simulink model "Appl_PaMemory_CtrlModel"  (R2018b)
settings: configuration reference "CodeConfig_10_ms" (kept outside this file)
undefined symbols (not defined in the file): CAL_PaMem_100MS, CAL_PaMem_90MS, D_ToleranceDistance, FALSE, TRUE
libraries: DareLib x89, simulink x1
(part 1 of 3)
settings Model: Creator=Administrator  LastModifiedBy=Administrator
settings ConfigSetRef: SourceLocation=Base Workspace

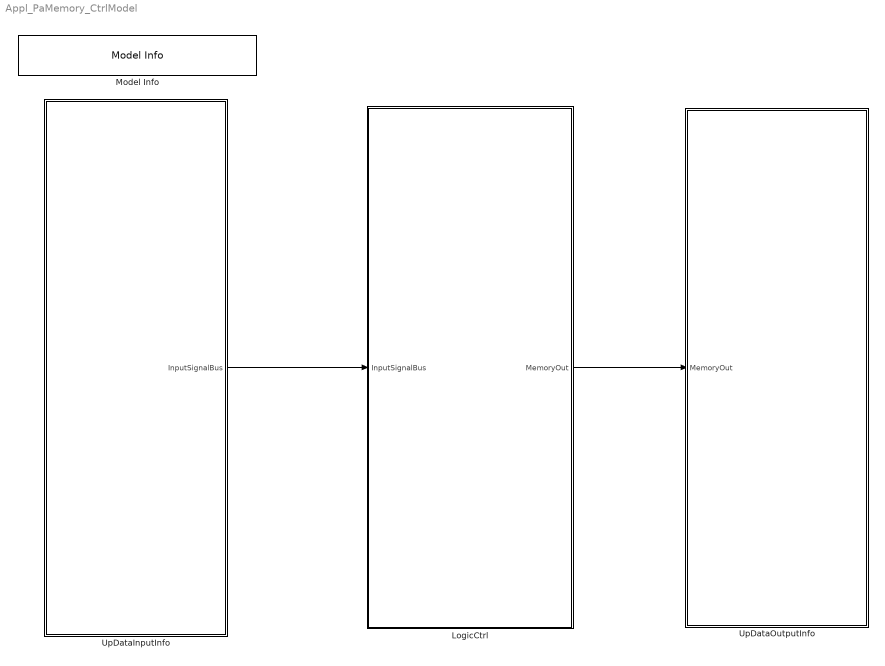
== system Appl_PaMemory_CtrlModel ==
  LogicCtrl : Subsystem  Priority=2  TreatAsAtomicUnit=on
      settings: RTWSystemCode=Nonreusable function  RTWFcnNameOpts=Use subsystem name
  Model Info : simulink/Model-Wide Utilities/Model Info  Frame=on  DisplayStringWithTags=Version：%<ModelVersion>  HorizontalTextAlignment=Center  LeftAlignmentValue=0.5
  UpDataInputInfo : Subsystem  Priority=1  TreatAsAtomicUnit=on
      settings: RTWSystemCode=Nonreusable function  RTWFcnNameOpts=Use subsystem name
  UpDataOutputInfo : Subsystem  Priority=3  TreatAsAtomicUnit=on
      settings: RTWSystemCode=Nonreusable function  RTWFcnNameOpts=Use subsystem name
  wires:
  LogicCtrl/1(MemoryOut) -> UpDataOutputInfo/1(MemoryOut)
  UpDataInputInfo/1(InputSignalBus) -> LogicCtrl/1(InputSignalBus)

== system Appl_PaMemory_CtrlModel/LogicCtrl ==
  InputSignalBus : Inport
  Bus Selector : BusSelector  OutputSignals=SeatMemBtn,CallMem,MemorySetPrecondition,MemoryRemindPrecondition,Rte_SignalBus.PaMem_HeightHallPosi,Rte_SignalBus.PaMem_LengthHallPosi,Rte_SignalBus.PaMem_BackHallPosi,Rte_SignalBus.PaMem_FrontHallPosi,Rte_SignalBus.PaMem_HeightAutoRunFlag,Rte_SignalBus.PaMem_LengthAutoRunFlag,Rte_SignalBus.PaMem_BackAutoRunFlag,Rte_SignalBus.PaMem_FrontAutoRunFlag,Rte_SignalBus.PaMem_AdjustEnable,Rte_SignalBus.PaMem_FRSeatPosMsg,Rte_SignalBus.PaMem_CurrentMoveType,Rte_SignalBus.PaMem_GetRecoverDefaultFlag,Rte_SignalBus.PaMem_HeightLockFault,Rte_SignalBus.PaMem_LengthLockFault,Rte_SignalBus.PaMem_BackLockFault,Rte_SignalBus.PaMem_FrontLockFault
  LocalAdjustCtrl : Subsystem  Description=加热逻辑处理
      settings: AttributesFormatString=%<Description>
  MainVent_OutputLvlSts : BusCreator  Inputs=13
  MemoryOut : Outport
  wires:
  InputSignalBus/1 -> Bus Selector/1  "InputSignalBus"
  MainVent_OutputLvlSts/1 -> MemoryOut/1  "MemoryOut"
  Bus Selector/1 -> LocalAdjustCtrl/1(SeatMemBtn)  "<SeatMemBtn>"
  Bus Selector/2 -> LocalAdjustCtrl/2(CallMem)  "<CallMem>"
  Bus Selector/3 -> LocalAdjustCtrl/3(MemorySetPrecondition)  "<MemorySetPrecondition>"
  Bus Selector/4 -> LocalAdjustCtrl/4(MemoryRemindPrecondition)  "<MemoryRemindPrecondition>"
  Bus Selector/5 -> LocalAdjustCtrl/5(PaMem_HeightHallPosi)  "<PaMem_HeightHallPosi>"
  Bus Selector/6 -> LocalAdjustCtrl/6(PaMem_LengthHallPosi)  "<PaMem_LengthHallPosi>"
  Bus Selector/7 -> LocalAdjustCtrl/7(PaMem_BackHallPosi)  "<PaMem_BackHallPosi>"
  Bus Selector/8 -> LocalAdjustCtrl/8(PaMem_FrontHallPosi)  "<PaMem_FrontHallPosi>"
  Bus Selector/9 -> LocalAdjustCtrl/9(PaMem_HeightAutoRunFlag)  "<PaMem_HeightAutoRunFlag>"
  Bus Selector/10 -> LocalAdjustCtrl/10(PaMem_LengthAutoRunFlag)  "<PaMem_LengthAutoRunFlag>"
  Bus Selector/11 -> LocalAdjustCtrl/11(PaMem_BackAutoRunFlag)  "<PaMem_BackAutoRunFlag>"
  Bus Selector/12 -> LocalAdjustCtrl/12(PaMem_FrontAutoRunFlag)  "<PaMem_FrontAutoRunFlag>"
  Bus Selector/13 -> LocalAdjustCtrl/13(PaMem_AdjustEnable)  "<PaMem_AdjustEnable>"
  Bus Selector/14 -> LocalAdjustCtrl/14(PaMem_FRSeatPosMsg)  "<PaMem_FRSeatPosMsg>"
  Bus Selector/15 -> LocalAdjustCtrl/15(PaMem_CurrentMoveType)  "<PaMem_CurrentMoveType>"
  Bus Selector/16 -> LocalAdjustCtrl/16(PaMem_GetRecoverDefaultFlag)  "<PaMem_GetRecoverDefaultFlag>"
  Bus Selector/17 -> LocalAdjustCtrl/17(PaMem_HeightLockFault)  "<PaMem_HeightLockFault>"
  Bus Selector/18 -> LocalAdjustCtrl/18(PaMem_LengthLockFault)  "<PaMem_LengthLockFault>"
  Bus Selector/19 -> LocalAdjustCtrl/19(PaMem_BackLockFault)  "<PaMem_BackLockFault>"
  Bus Selector/20 -> LocalAdjustCtrl/20(PaMem_FrontLockFault)  "<PaMem_FrontLockFault>"
  LocalAdjustCtrl/1(FRSeatMemSetSts) -> MainVent_OutputLvlSts/1
  LocalAdjustCtrl/2(MemSetStopReason) -> MainVent_OutputLvlSts/2
  LocalAdjustCtrl/3(FRSeatPosMsg) -> MainVent_OutputLvlSts/3
  LocalAdjustCtrl/4(SeatMemoryValidReq) -> MainVent_OutputLvlSts/4
  LocalAdjustCtrl/5(SeatHeightPosiReq) -> MainVent_OutputLvlSts/5
  LocalAdjustCtrl/6(SeatLengthPosiReq) -> MainVent_OutputLvlSts/6
  LocalAdjustCtrl/7(SeatBackPosiReq) -> MainVent_OutputLvlSts/7
  LocalAdjustCtrl/8(SeatFrontPosiReq) -> MainVent_OutputLvlSts/8
  LocalAdjustCtrl/9(MemCallStopReason) -> MainVent_OutputLvlSts/9
  LocalAdjustCtrl/10(SeatMem1StsFb) -> MainVent_OutputLvlSts/10
  LocalAdjustCtrl/11(SeatMem2StsFb) -> MainVent_OutputLvlSts/11
  LocalAdjustCtrl/12(SeatMem3StsFb) -> MainVent_OutputLvlSts/12
  LocalAdjustCtrl/13(PreMemRemindStop) -> MainVent_OutputLvlSts/13

== system Appl_PaMemory_CtrlModel/UpDataInputInfo ==
  InputSignalProcess : Subsystem  Description=数据处理
      settings: AttributesFormatString=%<Description>  RTWSystemCode=Nonreusable function  RTWFcnNameOpts=Use subsystem name
  RTE : Subsystem  Description=接口自动生成  TreatAsAtomicUnit=on
      settings: AttributesFormatString=%<Description>  RTWSystemCode=Nonreusable function  RTWFcnNameOpts=Use subsystem name
  InputSignalBus : Outport
  wires:
  RTE/1(RTE_Signal) -> InputSignalProcess/1(Rte_SignalBus)
  InputSignalProcess/1(InputSignalBus) -> InputSignalBus/1

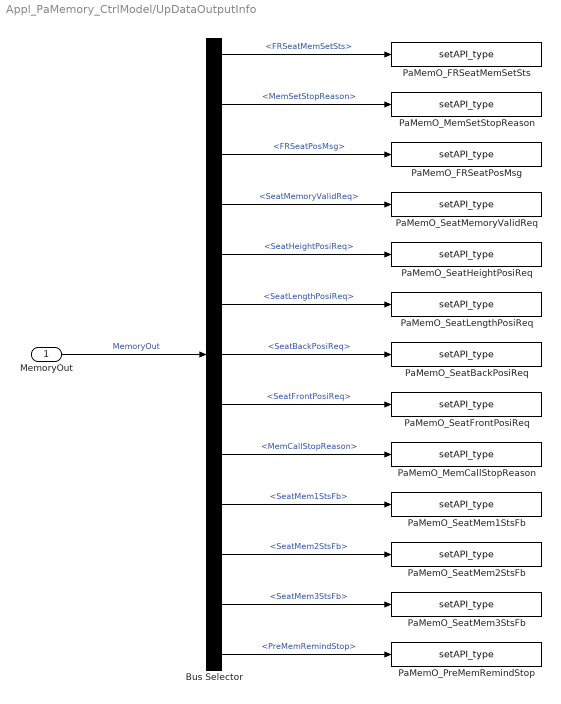
== system Appl_PaMemory_CtrlModel/UpDataOutputInfo ==
  MemoryOut : Inport
  Bus Selector : BusSelector  OutputSignals=FRSeatMemSetSts,MemSetStopReason,FRSeatPosMsg,SeatMemoryValidReq,SeatHeightPosiReq,SeatLengthPosiReq,SeatBackPosiReq,SeatFrontPosiReq,MemCallStopReason,SeatMem1StsFb,SeatMem2StsFb,SeatMem3StsFb,PreMemRemindStop
  PaMemO_FRSeatMemSetSts : DareLib/Dare/setAPI_type  g_funcname=CanTx_0x3B2_DSM_FRSeatMemStsAndMsg  g_param=""  g_type=uint8  g_enum=enMemSetFb  g_size=-1
      settings: AttributesFormatString=%<g_funcname>  SourceProductName=Dare Library
  PaMemO_FRSeatPosMsg : DareLib/Dare/setAPI_type  g_funcname=CanTx_0x3B2_DSM_FRSeatPosMsg  g_param=""  g_type=uint8  g_size=-1
      settings: AttributesFormatString=%<g_funcname>  SourceProductName=Dare Library
  PaMemO_MemCallStopReason : DareLib/Dare/setAPI_type  g_funcname=Rte_SetVfb_PaMemCallStopReason  g_param=""  g_type=uint8  g_enum=enMemStopCause  g_size=-1
      settings: AttributesFormatString=%<g_funcname>  SourceProductName=Dare Library
  PaMemO_MemSetStopReason : DareLib/Dare/setAPI_type  g_funcname=Rte_SetVfb_PaMemSetStopReason  g_param=""  g_type=uint8  g_enum=enMemStopCause  g_size=-1
      settings: AttributesFormatString=%<g_funcname>  SourceProductName=Dare Library
  PaMemO_PreMemRemindStop : DareLib/Dare/setAPI_type  g_funcname=Rte_SetVfb_PaPreMemRemindStop  g_param=""  g_type=uint8  g_enum=enMemStopCause  g_size=-1
      settings: AttributesFormatString=%<g_funcname>  SourceProductName=Dare Library
  PaMemO_SeatBackPosiReq : DareLib/Dare/setAPI_type  g_funcname=Rte_SetVfb_PaMemBackReqPosi  g_param=""  g_type=uint16  g_size=-1
      settings: AttributesFormatString=%<g_funcname>  SourceProductName=Dare Library
  PaMemO_SeatFrontPosiReq : DareLib/Dare/setAPI_type  g_funcname=Rte_SetVfb_PaMemFrontReqPosi  g_param=""  g_type=uint16  g_size=-1
      settings: AttributesFormatString=%<g_funcname>  SourceProductName=Dare Library
  PaMemO_SeatHeightPosiReq : DareLib/Dare/setAPI_type  g_funcname=Rte_SetVfb_PaMemHeightReqPosi  g_param=""  g_type=uint16  g_size=-1
      settings: AttributesFormatString=%<g_funcname>  SourceProductName=Dare Library
  PaMemO_SeatLengthPosiReq : DareLib/Dare/setAPI_type  g_funcname=Rte_SetVfb_PaMemLengthReqPosi  g_param=""  g_type=uint16  g_size=-1
      settings: AttributesFormatString=%<g_funcname>  SourceProductName=Dare Library
  PaMemO_SeatMem1StsFb : DareLib/Dare/setAPI_type  g_funcname=CanTx_0x3B2_DSM1_FRSeatMem1Sts  g_param=""  g_type=uint8  g_enum=enMemCallFb  g_size=-1
      settings: AttributesFormatString=%<g_funcname>  SourceProductName=Dare Library
  PaMemO_SeatMem2StsFb : DareLib/Dare/setAPI_type  g_funcname=CanTx_0x3B2_DSM2_FRSeatMem2Sts  g_param=""  g_type=uint8  g_enum=enMemCallFb  g_size=-1
      settings: AttributesFormatString=%<g_funcname>  SourceProductName=Dare Library
  PaMemO_SeatMem3StsFb : DareLib/Dare/setAPI_type  g_funcname=CanTx_0x3B2_DSM2_FRSeatMem3Sts  g_param=""  g_type=uint8  g_enum=enMemCallFb  g_size=-1
      settings: AttributesFormatString=%<g_funcname>  SourceProductName=Dare Library
  PaMemO_SeatMemoryValidReq : DareLib/Dare/setAPI_type  g_funcname=Rte_SetVfb_PaSeatMemoryValidReq  g_param=""  g_type=uint8  g_size=-1
      settings: AttributesFormatString=%<g_funcname>  SourceProductName=Dare Library
  wires:
  MemoryOut/1 -> Bus Selector/1  "MemoryOut"
  Bus Selector/2 -> PaMemO_MemSetStopReason/1  "<MemSetStopReason>"
  Bus Selector/1 -> PaMemO_FRSeatMemSetSts/1  "<FRSeatMemSetSts>"
  Bus Selector/3 -> PaMemO_FRSeatPosMsg/1  "<FRSeatPosMsg>"
  Bus Selector/4 -> PaMemO_SeatMemoryValidReq/1  "<SeatMemoryValidReq>"
  Bus Selector/5 -> PaMemO_SeatHeightPosiReq/1  "<SeatHeightPosiReq>"
  Bus Selector/6 -> PaMemO_SeatLengthPosiReq/1  "<SeatLengthPosiReq>"
  Bus Selector/7 -> PaMemO_SeatBackPosiReq/1  "<SeatBackPosiReq>"
  Bus Selector/8 -> PaMemO_SeatFrontPosiReq/1  "<SeatFrontPosiReq>"
  Bus Selector/9 -> PaMemO_MemCallStopReason/1  "<MemCallStopReason>"
  Bus Selector/10 -> PaMemO_SeatMem1StsFb/1  "<SeatMem1StsFb>"
  Bus Selector/11 -> PaMemO_SeatMem2StsFb/1  "<SeatMem2StsFb>"
  Bus Selector/12 -> PaMemO_SeatMem3StsFb/1  "<SeatMem3StsFb>"
  Bus Selector/13 -> PaMemO_PreMemRemindStop/1  "<PreMemRemindStop>"

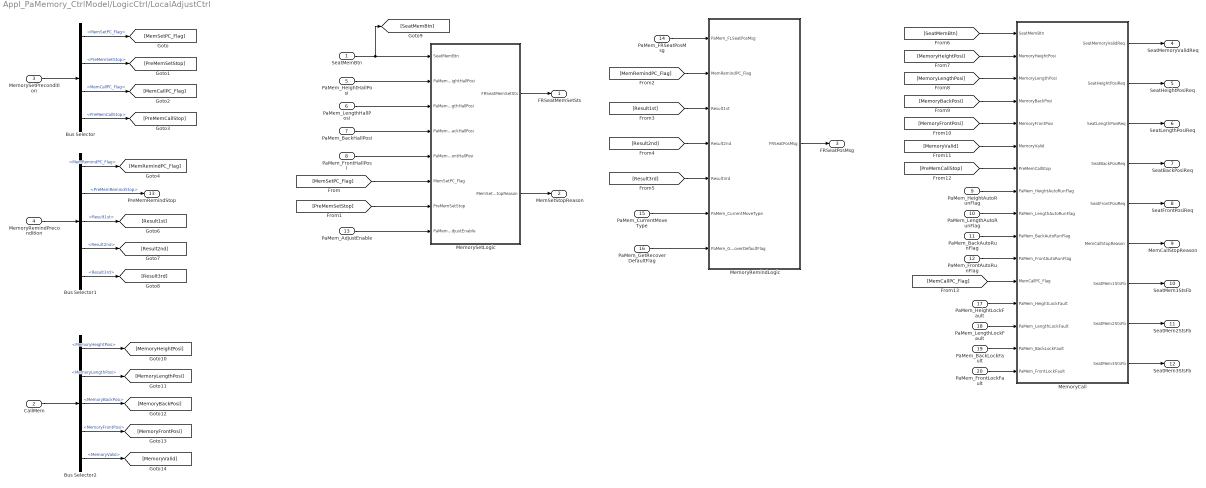
== system Appl_PaMemory_CtrlModel/LogicCtrl/LocalAdjustCtrl ==
  SeatMemBtn : Inport
  CallMem : Inport  Port=2
  MemorySetPrecondition : Inport  Port=3
  MemoryRemindPrecondition : Inport  Port=4
  PaMem_HeightHallPosi : Inport  Port=5
  PaMem_LengthHallPosi : Inport  Port=6
  PaMem_BackHallPosi : Inport  Port=7
  PaMem_FrontHallPosi : Inport  Port=8
  PaMem_HeightAutoRunFlag : Inport  Port=9
  PaMem_LengthAutoRunFlag : Inport  Port=10
  PaMem_BackAutoRunFlag : Inport  Port=11
  PaMem_FrontAutoRunFlag : Inport  Port=12
  PaMem_AdjustEnable : Inport  Port=13
  PaMem_FRSeatPosMsg : Inport  Port=14
  PaMem_CurrentMoveType : Inport  Port=15
  PaMem_GetRecoverDefaultFlag : Inport  Port=16
  PaMem_HeightLockFault : Inport  Port=17
  PaMem_LengthLockFault : Inport  Port=18
  PaMem_BackLockFault : Inport  Port=19
  PaMem_FrontLockFault : Inport  Port=20
  Bus Selector : BusSelector  OutputSignals=MemSetPC_Flag,PreMemSetStop,MemCallPC_Flag,PreMemCallStop
  Bus Selector1 : BusSelector  OutputSignals=MemRemindPC_Flag,PreMemRemindStop,Result1st,Result2nd,Result3rd
  Bus Selector2 : BusSelector  OutputSignals=MemoryHeightPosi,MemoryLengthPosi,MemoryBackPosi,MemoryFrontPosi,MemoryValid
  MemoryCall : Stateflow chart  TreatAsAtomicUnit=on
  MemoryRemindLogic : Stateflow chart  TreatAsAtomicUnit=on
  MemorySetLogic : Stateflow chart  TreatAsAtomicUnit=on
  FRSeatMemSetSts : Outport
  MemSetStopReason : Outport  Port=2
  FRSeatPosMsg : Outport  Port=3
  SeatMemoryValidReq : Outport  Port=4
  SeatHeightPosiReq : Outport  Port=5
  SeatLengthPosiReq : Outport  Port=6
  SeatBackPosiReq : Outport  Port=7
  SeatFrontPosiReq : Outport  Port=8
  MemCallStopReason : Outport  Port=9
  SeatMem1StsFb : Outport  Port=10
  SeatMem2StsFb : Outport  Port=11
  SeatMem3StsFb : Outport  Port=12
  PreMemRemindStop : Outport  Port=13
  wires:
  SeatMemBtn/1 -> [SeatMemBtn], MemorySetLogic/1(SeatMemBtn)
  PaMem_HeightHallPosi/1 -> MemorySetLogic/2(PaMem_HeightHallPosi)
  PaMem_LengthHallPosi/1 -> MemorySetLogic/3(PaMem_LengthHallPosi)
  PaMem_BackHallPosi/1 -> MemorySetLogic/4(PaMem_BackHallPosi)
  PaMem_FrontHallPosi/1 -> MemorySetLogic/5(PaMem_FrontHallPosi)
  MemorySetPrecondition/1 -> Bus Selector/1
  Bus Selector/1 -> [MemSetPC_Flag]  "<MemSetPC_Flag>"
  Bus Selector/2 -> [PreMemSetStop]  "<PreMemSetStop>"
  Bus Selector/3 -> [MemCallPC_Flag]  "<MemCallPC_Flag>"
  Bus Selector/4 -> [PreMemCallStop]  "<PreMemCallStop>"
  [MemSetPC_Flag] -> MemorySetLogic/6(MemSetPC_Flag)
  [PreMemSetStop] -> MemorySetLogic/7(PreMemSetStop)
  PaMem_AdjustEnable/1 -> MemorySetLogic/8(PaMem_AdjustEnable)
  MemoryRemindPrecondition/1 -> Bus Selector1/1
  Bus Selector1/4 -> [Result2nd]  "<Result2nd>"
  Bus Selector1/3 -> [Result1st]  "<Result1st>"
  Bus Selector1/5 -> [Result3rd]  "<Result3rd>"
  Bus Selector1/1 -> [MemRemindPC_Flag]  "<MemRemindPC_Flag>"
  PaMem_FRSeatPosMsg/1 -> MemoryRemindLogic/1(PaMem_FLSeatPosMsg)
  [MemRemindPC_Flag] -> MemoryRemindLogic/2(MemRemindPC_Flag)
  [Result1st] -> MemoryRemindLogic/3(Result1st)
  [Result2nd] -> MemoryRemindLogic/4(Result2nd)
  [Result3rd] -> MemoryRemindLogic/5(Result3rd)
  PaMem_CurrentMoveType/1 -> MemoryRemindLogic/6(PaMem_CurrentMoveType)
  PaMem_GetRecoverDefaultFlag/1 -> MemoryRemindLogic/7(PaMem_GetRecoverDefaultFlag)
  CallMem/1 -> Bus Selector2/1
  Bus Selector2/1 -> [MemoryHeightPosi]  "<MemoryHeightPosi>"
  Bus Selector2/2 -> [MemoryLengthPosi]  "<MemoryLengthPosi>"
  Bus Selector2/3 -> [MemoryBackPosi]  "<MemoryBackPosi>"
  Bus Selector2/4 -> [MemoryFrontPosi]  "<MemoryFrontPosi>"
  Bus Selector2/5 -> [MemoryValid]  "<MemoryValid>"
  [SeatMemBtn] -> MemoryCall/1(SeatMemBtn)
  [MemoryHeightPosi] -> MemoryCall/2(MemoryHeightPosi)
  [MemoryLengthPosi] -> MemoryCall/3(MemoryLengthPosi)
  [MemoryBackPosi] -> MemoryCall/4(MemoryBackPosi)
  [MemoryFrontPosi] -> MemoryCall/5(MemoryFrontPosi)
  [MemoryValid] -> MemoryCall/6(MemoryValid)
  [PreMemCallStop] -> MemoryCall/7(PreMemCallStop)
  PaMem_HeightAutoRunFlag/1 -> MemoryCall/8(PaMem_HeightAutoRunFlag)
  PaMem_LengthAutoRunFlag/1 -> MemoryCall/9(PaMem_LengthAutoRunFlag)
  PaMem_BackAutoRunFlag/1 -> MemoryCall/10(PaMem_BackAutoRunFlag)
  PaMem_FrontAutoRunFlag/1 -> MemoryCall/11(PaMem_FrontAutoRunFlag)
  [MemCallPC_Flag] -> MemoryCall/12(MemCallPC_Flag)
  PaMem_FrontLockFault/1 -> MemoryCall/16(PaMem_FrontLockFault)
  PaMem_BackLockFault/1 -> MemoryCall/15(PaMem_BackLockFault)
  PaMem_LengthLockFault/1 -> MemoryCall/14(PaMem_LengthLockFault)
  PaMem_HeightLockFault/1 -> MemoryCall/13(PaMem_HeightLockFault)
  MemorySetLogic/1(FRSeatMemSetSts) -> FRSeatMemSetSts/1
  MemorySetLogic/2(MemSetStopReason) -> MemSetStopReason/1
  MemoryRemindLogic/1(FRSeatPosMsg) -> FRSeatPosMsg/1
  MemoryCall/1(SeatMemoryValidReq) -> SeatMemoryValidReq/1
  MemoryCall/2(SeatHeightPosiReq) -> SeatHeightPosiReq/1
  MemoryCall/3(SeatLengthPosiReq) -> SeatLengthPosiReq/1
  MemoryCall/4(SeatBackPosiReq) -> SeatBackPosiReq/1
  MemoryCall/5(SeatFrontPosiReq) -> SeatFrontPosiReq/1
  MemoryCall/6(MemCallStopReason) -> MemCallStopReason/1
  MemoryCall/7(SeatMem1StsFb) -> SeatMem1StsFb/1
  MemoryCall/8(SeatMem2StsFb) -> SeatMem2StsFb/1
  MemoryCall/9(SeatMem3StsFb) -> SeatMem3StsFb/1
  Bus Selector1/2 -> PreMemRemindStop/1  "<PreMemRemindStop>"

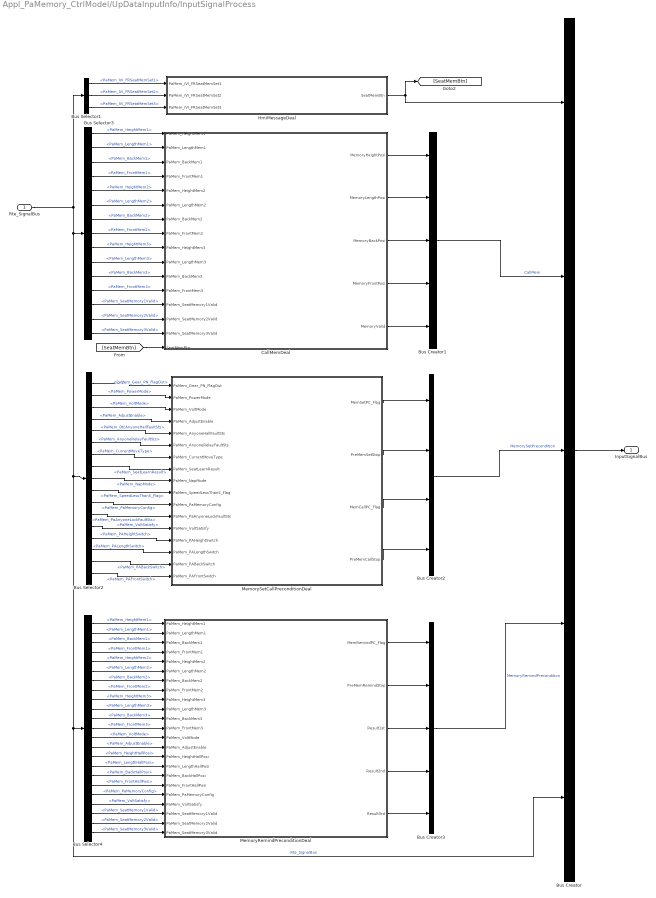
== system Appl_PaMemory_CtrlModel/UpDataInputInfo/InputSignalProcess ==
  Rte_SignalBus : Inport
  Bus Creator : BusCreator  Inputs=5
  Bus Creator1 : BusCreator  Inputs=5
  Bus Creator2 : BusCreator  Inputs=4
  Bus Creator3 : BusCreator  Inputs=5
  Bus Selector1 : BusSelector  OutputSignals=PaMem_IVI_FRSeatMemSet1,PaMem_IVI_FRSeatMemSet2,PaMem_IVI_FRSeatMemSet3
  Bus Selector2 : BusSelector  OutputSignals=PaMem_Gear_PN_FlagOut,PaMem_PowerMode,PaMem_VoltMode,PaMem_AdjustEnable,PaMem_DtcAnyoneHallFaultSts,PaMem_AnyoneRelayFaultSts,PaMem_CurrentMoveType,PaMem_SeatLearnResult,PaMem_NapMode,PaMem_SpeedLessThan5_Flag,PaMem_PaMemoryConfig,PaMem_PaAnyoneLockFaultSts,PaMem_VoltSatisfy,PaMem_PAHeightSwitch,PaMem_PALengthSwitch,PaMem_PABackSwitch,PaMem_PAFrontSwitch
  Bus Selector3 : BusSelector  OutputSignals=PaMem_HeightMem1,PaMem_LengthMem1,PaMem_BackMem1,PaMem_FrontMem1,PaMem_HeightMem2,PaMem_LengthMem2,PaMem_BackMem2,PaMem_FrontMem2,PaMem_HeightMem3,PaMem_LengthMem3,PaMem_BackMem3,PaMem_FrontMem3,PaMem_SeatMemory1Valid,PaMem_SeatMemory2Valid,PaMem_SeatMemory3Valid
  Bus Selector4 : BusSelector  OutputSignals=PaMem_HeightMem1,PaMem_LengthMem1,PaMem_BackMem1,PaMem_FrontMem1,PaMem_HeightMem2,PaMem_LengthMem2,PaMem_BackMem2,PaMem_FrontMem2,PaMem_HeightMem3,PaMem_LengthMem3,PaMem_BackMem3,PaMem_FrontMem3,PaMem_VoltMode,PaMem_AdjustEnable,PaMem_HeightHallPosi,PaMem_LengthHallPosi,PaMem_BackHallPosi,PaMem_FrontHallPosi,PaMem_PaMemoryConfig,PaMem_VoltSatisfy,PaMem_SeatMemory1Valid,PaMem_SeatMemory2Valid,PaMem_SeatMemory3Valid
  CallMemDeal : Subsystem  Description=记忆调用位置处理
      settings: AttributesFormatString=%<Description>
  HmiMessageDeal : Subsystem  Description=记忆报文处理
      settings: AttributesFormatString=%<Description>
  MemoryRemindPreconditionDeal : Subsystem  Description=记忆提示前置条件处理
      settings: AttributesFormatString=%<Description>
  MemorySetCallPreconditionDeal : Subsystem  Description=记忆设置与调用前置条件处理
      settings: AttributesFormatString=%<Description>
  InputSignalBus : Outport
  wires:
  Bus Creator/1 -> InputSignalBus/1
  Rte_SignalBus/1 -> Bus Selector4/1, Bus Creator/5, Bus Selector2/1, Bus Selector3/1, Bus Selector1/1  "Rte_SignalBus"
  HmiMessageDeal/1(SeatMemBtn) -> [SeatMemBtn], Bus Creator/1
  Bus Selector1/1 -> HmiMessageDeal/1(PaMem_IVI_FRSeatMemSet1)  "<PaMem_IVI_FRSeatMemSet1>"
  Bus Selector1/2 -> HmiMessageDeal/2(PaMem_IVI_FRSeatMemSet2)  "<PaMem_IVI_FRSeatMemSet2>"
  Bus Selector1/3 -> HmiMessageDeal/3(PaMem_IVI_FRSeatMemSet3)  "<PaMem_IVI_FRSeatMemSet3>"
  Bus Selector3/1 -> CallMemDeal/1(PaMem_HeightMem1)  "<PaMem_HeightMem1>"
  Bus Selector3/2 -> CallMemDeal/2(PaMem_LengthMem1)  "<PaMem_LengthMem1>"
  Bus Selector3/3 -> CallMemDeal/3(PaMem_BackMem1)  "<PaMem_BackMem1>"
  Bus Selector3/4 -> CallMemDeal/4(PaMem_FrontMem1)  "<PaMem_FrontMem1>"
  Bus Selector3/5 -> CallMemDeal/5(PaMem_HeightMem2)  "<PaMem_HeightMem2>"
  Bus Selector3/6 -> CallMemDeal/6(PaMem_LengthMem2)  "<PaMem_LengthMem2>"
  Bus Selector3/7 -> CallMemDeal/7(PaMem_BackMem2)  "<PaMem_BackMem2>"
  Bus Selector3/8 -> CallMemDeal/8(PaMem_FrontMem2)  "<PaMem_FrontMem2>"
  Bus Selector3/9 -> CallMemDeal/9(PaMem_HeightMem3)  "<PaMem_HeightMem3>"
  Bus Selector3/10 -> CallMemDeal/10(PaMem_LengthMem3)  "<PaMem_LengthMem3>"
  Bus Selector3/11 -> CallMemDeal/11(PaMem_BackMem3)  "<PaMem_BackMem3>"
  Bus Selector3/12 -> CallMemDeal/12(PaMem_FrontMem3)  "<PaMem_FrontMem3>"
  [SeatMemBtn] -> CallMemDeal/16(SeatMemBtn)
  CallMemDeal/1(MemoryHeightPosi) -> Bus Creator1/1
  CallMemDeal/2(MemoryLengthPosi) -> Bus Creator1/2
  CallMemDeal/3(MemoryBackPosi) -> Bus Creator1/3
  CallMemDeal/4(MemoryFrontPosi) -> Bus Creator1/4
  CallMemDeal/5(MemoryValid) -> Bus Creator1/5
  Bus Selector2/2 -> MemorySetCallPreconditionDeal/2(PaMem_PowerMode)  "<PaMem_PowerMode>"
  Bus Selector2/1 -> MemorySetCallPreconditionDeal/1(PaMem_Gear_PN_FlagOut)  "<PaMem_Gear_PN_FlagOut>"
  Bus Selector2/3 -> MemorySetCallPreconditionDeal/3(PaMem_VoltMode)  "<PaMem_VoltMode>"
  Bus Selector2/4 -> MemorySetCallPreconditionDeal/4(PaMem_AdjustEnable)  "<PaMem_AdjustEnable>"
  Bus Selector2/5 -> MemorySetCallPreconditionDeal/5(PaMem_AnyoneHallFaultSts)  "<PaMem_DtcAnyoneHallFaultSts>"
  Bus Selector2/7 -> MemorySetCallPreconditionDeal/7(PaMem_CurrentMoveType)  "<PaMem_CurrentMoveType>"
  Bus Selector2/8 -> MemorySetCallPreconditionDeal/8(PaMem_SeatLearnResult)  "<PaMem_SeatLearnResult>"
  Bus Selector2/9 -> MemorySetCallPreconditionDeal/9(PaMem_NapMode)  "<PaMem_NapMode>"
  Bus Selector2/6 -> MemorySetCallPreconditionDeal/6(PaMem_AnyoneRelayFaultSts)  "<PaMem_AnyoneRelayFaultSts>"
  Bus Selector4/5 -> MemoryRemindPreconditionDeal/5(PaMem_HeightMem2)  "<PaMem_HeightMem2>"
  Bus Selector4/4 -> MemoryRemindPreconditionDeal/4(PaMem_FrontMem1)  "<PaMem_FrontMem1>"
  Bus Selector4/6 -> MemoryRemindPreconditionDeal/6(PaMem_LengthMem2)  "<PaMem_LengthMem2>"
  Bus Selector4/3 -> MemoryRemindPreconditionDeal/3(PaMem_BackMem1)  "<PaMem_BackMem1>"
  Bus Selector4/7 -> MemoryRemindPreconditionDeal/7(PaMem_BackMem2)  "<PaMem_BackMem2>"
  Bus Selector4/2 -> MemoryRemindPreconditionDeal/2(PaMem_LengthMem1)  "<PaMem_LengthMem1>"
  Bus Selector4/8 -> MemoryRemindPreconditionDeal/8(PaMem_FrontMem2)  "<PaMem_FrontMem2>"
  Bus Selector4/1 -> MemoryRemindPreconditionDeal/1(PaMem_HeightMem1)  "<PaMem_HeightMem1>"
  Bus Selector4/9 -> MemoryRemindPreconditionDeal/9(PaMem_HeightMem3)  "<PaMem_HeightMem3>"
  Bus Selector4/10 -> MemoryRemindPreconditionDeal/10(PaMem_LengthMem3)  "<PaMem_LengthMem3>"
  Bus Selector4/11 -> MemoryRemindPreconditionDeal/11(PaMem_BackMem3)  "<PaMem_BackMem3>"
  Bus Selector4/12 -> MemoryRemindPreconditionDeal/12(PaMem_FrontMem3)  "<PaMem_FrontMem3>"
  Bus Selector4/13 -> MemoryRemindPreconditionDeal/13(PaMem_VoltMode)  "<PaMem_VoltMode>"
  Bus Selector4/14 -> MemoryRemindPreconditionDeal/14(PaMem_AdjustEnable)  "<PaMem_AdjustEnable>"
  Bus Selector4/15 -> MemoryRemindPreconditionDeal/15(PaMem_HeightHallPosi)  "<PaMem_HeightHallPosi>"
  Bus Selector4/16 -> MemoryRemindPreconditionDeal/16(PaMem_LengthHallPosi)  "<PaMem_LengthHallPosi>"
  Bus Selector4/17 -> MemoryRemindPreconditionDeal/17(PaMem_BackHallPosi)  "<PaMem_BackHallPosi>"
  Bus Selector4/18 -> MemoryRemindPreconditionDeal/18(PaMem_FrontHallPosi)  "<PaMem_FrontHallPosi>"
  MemorySetCallPreconditionDeal/1(MemSetPC_Flag) -> Bus Creator2/1
  MemorySetCallPreconditionDeal/2(PreMemSetStop) -> Bus Creator2/2
  MemorySetCallPreconditionDeal/3(MemCallPC_Flag) -> Bus Creator2/3
  MemorySetCallPreconditionDeal/4(PreMemCallStop) -> Bus Creator2/4
  MemoryRemindPreconditionDeal/2(PreMemRemindStop) -> Bus Creator3/2
  MemoryRemindPreconditionDeal/1(MemRemindPC_Flag) -> Bus Creator3/1
  MemoryRemindPreconditionDeal/3(Result1st) -> Bus Creator3/3
  MemoryRemindPreconditionDeal/4(Result2nd) -> Bus Creator3/4
  MemoryRemindPreconditionDeal/5(Result3rd) -> Bus Creator3/5
  Bus Creator1/1 -> Bus Creator/2  "CallMem"
  Bus Creator2/1 -> Bus Creator/3  "MemorySetPrecondition"
  Bus Creator3/1 -> Bus Creator/4  "MemoryRemindPrecondition"
  Bus Selector3/13 -> CallMemDeal/13(PaMem_SeatMemory1Valid)  "<PaMem_SeatMemory1Valid>"
  Bus Selector3/14 -> CallMemDeal/14(PaMem_SeatMemory2Valid)  "<PaMem_SeatMemory2Valid>"
  Bus Selector3/15 -> CallMemDeal/15(PaMem_SeatMemory3Valid)  "<PaMem_SeatMemory3Valid>"
  Bus Selector2/10 -> MemorySetCallPreconditionDeal/10(PaMem_SpeedLessThan5_Flag)  "<PaMem_SpeedLessThan5_Flag>"
  Bus Selector2/11 -> MemorySetCallPreconditionDeal/11(PaMem_PaMemoryConfig)  "<PaMem_PaMemoryConfig>"
  Bus Selector4/19 -> MemoryRemindPreconditionDeal/19(PaMem_PaMemoryConfig)  "<PaMem_PaMemoryConfig>"
  Bus Selector2/12 -> MemorySetCallPreconditionDeal/12(PaMem_PaAnyoneLockFaultSts)  "<PaMem_PaAnyoneLockFaultSts>"
  Bus Selector2/13 -> MemorySetCallPreconditionDeal/13(PaMem_VoltSatisfy)  "<PaMem_VoltSatisfy>"
  Bus Selector4/20 -> MemoryRemindPreconditionDeal/20(PaMem_VoltSatisfy)  "<PaMem_VoltSatisfy>"
  Bus Selector4/21 -> MemoryRemindPreconditionDeal/21(PaMem_SeatMemory1Valid)  "<PaMem_SeatMemory1Valid>"
  Bus Selector4/22 -> MemoryRemindPreconditionDeal/22(PaMem_SeatMemory2Valid)  "<PaMem_SeatMemory2Valid>"
  Bus Selector4/23 -> MemoryRemindPreconditionDeal/23(PaMem_SeatMemory3Valid)  "<PaMem_SeatMemory3Valid>"
  Bus Selector2/14 -> MemorySetCallPreconditionDeal/14(PaMem_PAHeightSwitch)  "<PaMem_PAHeightSwitch>"
  Bus Selector2/15 -> MemorySetCallPreconditionDeal/15(PaMem_PALengthSwitch)  "<PaMem_PALengthSwitch>"
  Bus Selector2/16 -> MemorySetCallPreconditionDeal/16(PaMem_PABackSwitch)  "<PaMem_PABackSwitch>"
  Bus Selector2/17 -> MemorySetCallPreconditionDeal/17(PaMem_PAFrontSwitch)  "<PaMem_PAFrontSwitch>"

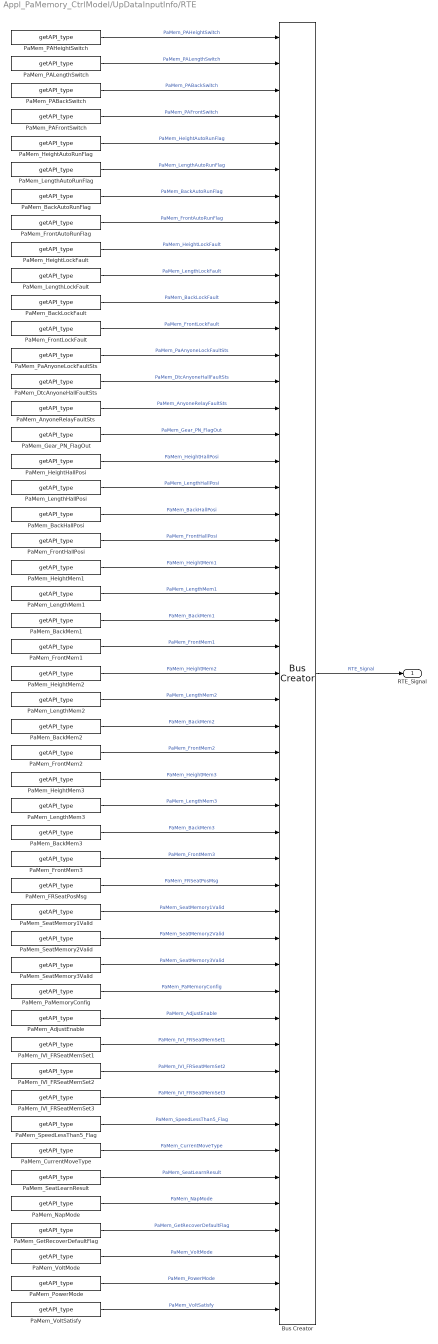
== system Appl_PaMemory_CtrlModel/UpDataInputInfo/RTE ==
  Bus Creator : BusCreator  Inputs=49
  PaMem_AdjustEnable : DareLib/Dare/getAPI_type  g_funcname=Srvl_GetMemIndexDataU8  g_param=EN_MemIndex_PaAdjustConfig  g_type=uint8  g_size=-1
      settings: AttributesFormatString=%<g_funcname>  SourceProductName=Dare Library
  PaMem_AnyoneRelayFaultSts : DareLib/Dare/getAPI_type  g_funcname=Rte_GetVfb_PaAnyoneRelayAdheErr  g_param=""  g_type=uint8  g_enum=enSeatMotorRunType  g_size=-1
      settings: AttributesFormatString=%<g_funcname>  SourceProductName=Dare Library
  PaMem_BackAutoRunFlag : DareLib/Dare/getAPI_type  g_funcname=Rte_GetVfb_PaBackAutoRunFlag  g_param=""  g_type=uint8  g_enum=enSeatAutoRunSts  g_size=-1
      settings: AttributesFormatString=%<g_funcname>  SourceProductName=Dare Library
  PaMem_BackHallPosi : DareLib/Dare/getAPI_type  g_funcname=Cdd_GetCurrentHallCnt  g_param=EN_PassengerBack  g_type=uint16  g_size=-1
      settings: AttributesFormatString=%<g_funcname>  SourceProductName=Dare Library
  PaMem_BackLockFault : DareLib/Dare/getAPI_type  g_funcname=Rte_GetVfb_PaBackStallErr  g_param=""  g_type=uint8  g_size=-1
      settings: AttributesFormatString=%<g_funcname>  SourceProductName=Dare Library
  PaMem_BackMem1 : DareLib/Dare/getAPI_type  g_funcname=Srvl_GetMemIndexDataU16  g_param=EN_MemIndex_PaMem1_Back  g_type=uint16  g_size=-1
      settings: AttributesFormatString=%<g_funcname>  SourceProductName=Dare Library
  PaMem_BackMem2 : DareLib/Dare/getAPI_type  g_funcname=Srvl_GetMemIndexDataU16  g_param=EN_MemIndex_PaMem2_Back  g_type=uint16  g_size=-1
      settings: AttributesFormatString=%<g_funcname>  SourceProductName=Dare Library
  PaMem_BackMem3 : DareLib/Dare/getAPI_type  g_funcname=Srvl_GetMemIndexDataU16  g_param=EN_MemIndex_PaMem3_Back  g_type=uint16  g_size=-1
      settings: AttributesFormatString=%<g_funcname>  SourceProductName=Dare Library
  PaMem_CurrentMoveType : DareLib/Dare/getAPI_type  g_funcname=Rte_GetVfb_PaMoveType  g_param=""  g_type=uint8  g_size=-1
      settings: AttributesFormatString=%<g_funcname>  SourceProductName=Dare Library
  PaMem_DtcAnyoneHallFaultSts : DareLib/Dare/getAPI_type  g_funcname=Rte_GetVfb_PaAnyoneDTCHallErr  g_param=""  g_type=uint8  g_size=-1
      settings: AttributesFormatString=%<g_funcname>  SourceProductName=Dare Library
  PaMem_FRSeatPosMsg : DareLib/Dare/getAPI_type  g_funcname=Srvl_GetMemIndexDataU8  g_param=EN_MemIndex_FRSeatPosMsg  g_type=uint8  g_size=-1
      settings: AttributesFormatString=%<g_funcname>  SourceProductName=Dare Library
  PaMem_FrontAutoRunFlag : DareLib/Dare/getAPI_type  g_funcname=Rte_GetVfb_PaFrontAutoRunFlag  g_param=""  g_type=uint8  g_enum=enSeatAutoRunSts  g_size=-1
      settings: AttributesFormatString=%<g_funcname>  SourceProductName=Dare Library
  PaMem_FrontHallPosi : DareLib/Dare/getAPI_type  g_funcname=Cdd_GetCurrentHallCnt  g_param=EN_PaResever_2  g_type=uint16  g_size=-1
      settings: AttributesFormatString=%<g_funcname>  SourceProductName=Dare Library
  PaMem_FrontLockFault : DareLib/Dare/getAPI_type  g_funcname=Rte_GetVfb_PaFrontStallErr  g_param=""  g_type=uint8  g_size=-1
      settings: AttributesFormatString=%<g_funcname>  SourceProductName=Dare Library
  PaMem_FrontMem1 : DareLib/Dare/getAPI_type  g_funcname=Srvl_GetMemIndexDataU16  g_param=EN_MemIndex_PaMem1_Front  g_type=uint16  g_size=-1
      settings: AttributesFormatString=%<g_funcname>  SourceProductName=Dare Library
  PaMem_FrontMem2 : DareLib/Dare/getAPI_type  g_funcname=Srvl_GetMemIndexDataU16  g_param=EN_MemIndex_PaMem2_Front  g_type=uint16  g_size=-1
      settings: AttributesFormatString=%<g_funcname>  SourceProductName=Dare Library
  PaMem_FrontMem3 : DareLib/Dare/getAPI_type  g_funcname=Srvl_GetMemIndexDataU16  g_param=EN_MemIndex_PaMem3_Front  g_type=uint16  g_size=-1
      settings: AttributesFormatString=%<g_funcname>  SourceProductName=Dare Library
  PaMem_Gear_PN_FlagOut : DareLib/Dare/getAPI_type  g_funcname=Rte_GetCAN_Gear_PN_Flag  g_param=""  g_type=uint8  g_size=-1
      settings: AttributesFormatString=%<g_funcname>  SourceProductName=Dare Library
  PaMem_GetRecoverDefaultFlag : DareLib/Dare/getAPI_type  g_funcname=GetRecoverDefaultFlag  g_param=""  g_type=uint16  g_size=-1
      settings: AttributesFormatString=%<g_funcname>  SourceProductName=Dare Library
  PaMem_HeightAutoRunFlag : DareLib/Dare/getAPI_type  g_funcname=Rte_GetVfb_PaHeightAutoRunFlag  g_param=""  g_type=uint8  g_enum=enSeatAutoRunSts  g_size=-1
      settings: AttributesFormatString=%<g_funcname>  SourceProductName=Dare Library
  PaMem_HeightHallPosi : DareLib/Dare/getAPI_type  g_funcname=Cdd_GetCurrentHallCnt  g_param=EN_PaResever_1  g_type=uint16  g_size=-1
      settings: AttributesFormatString=%<g_funcname>  SourceProductName=Dare Library
  PaMem_HeightLockFault : DareLib/Dare/getAPI_type  g_funcname=Rte_GetVfb_PaHeightStallErr  g_param=""  g_type=uint8  g_size=-1
      settings: AttributesFormatString=%<g_funcname>  SourceProductName=Dare Library
  PaMem_HeightMem1 : DareLib/Dare/getAPI_type  g_funcname=Srvl_GetMemIndexDataU16  g_param=EN_MemIndex_PaMem1_Height  g_type=uint16  g_size=-1
      settings: AttributesFormatString=%<g_funcname>  SourceProductName=Dare Library
  PaMem_HeightMem2 : DareLib/Dare/getAPI_type  g_funcname=Srvl_GetMemIndexDataU16  g_param=EN_MemIndex_PaMem2_Height  g_type=uint16  g_size=-1
      settings: AttributesFormatString=%<g_funcname>  SourceProductName=Dare Library
  PaMem_HeightMem3 : DareLib/Dare/getAPI_type  g_funcname=Srvl_GetMemIndexDataU16  g_param=EN_MemIndex_PaMem3_Height  g_type=uint16  g_size=-1
      settings: AttributesFormatString=%<g_funcname>  SourceProductName=Dare Library
  PaMem_IVI_FRSeatMemSet1 : DareLib/Dare/getAPI_type  g_funcname=CanRx_0x351_IVI_FRSeatMemSet1  g_param=""  g_type=uint8  g_enum=enMemSet  g_size=-1
      settings: AttributesFormatString=%<g_funcname>  SourceProductName=Dare Library
  PaMem_IVI_FRSeatMemSet2 : DareLib/Dare/getAPI_type  g_funcname=CanRx_0x351_IVI_FRSeatMemSet2  g_param=""  g_type=uint8  g_enum=enMemSet  g_size=-1
      settings: AttributesFormatString=%<g_funcname>  SourceProductName=Dare Library
  PaMem_IVI_FRSeatMemSet3 : DareLib/Dare/getAPI_type  g_funcname=CanRx_0x351_IVI_FRSeatMemSet3  g_param=""  g_type=uint8  g_enum=enMemSet  g_size=-1
      settings: AttributesFormatString=%<g_funcname>  SourceProductName=Dare Library
  PaMem_LengthAutoRunFlag : DareLib/Dare/getAPI_type  g_funcname=Rte_GetVfb_PaLengthAutoRunFlag  g_param=""  g_type=uint8  g_enum=enSeatAutoRunSts  g_size=-1
      settings: AttributesFormatString=%<g_funcname>  SourceProductName=Dare Library
  PaMem_LengthHallPosi : DareLib/Dare/getAPI_type  g_funcname=Cdd_GetCurrentHallCnt  g_param=EN_PassengerLength  g_type=uint16  g_size=-1
      settings: AttributesFormatString=%<g_funcname>  SourceProductName=Dare Library
  PaMem_LengthLockFault : DareLib/Dare/getAPI_type  g_funcname=Rte_GetVfb_PaLengthStallErr  g_param=""  g_type=uint8  g_size=-1
      settings: AttributesFormatString=%<g_funcname>  SourceProductName=Dare Library
  PaMem_LengthMem1 : DareLib/Dare/getAPI_type  g_funcname=Srvl_GetMemIndexDataU16  g_param=EN_MemIndex_PaMem1_Length  g_type=uint16  g_size=-1
      settings: AttributesFormatString=%<g_funcname>  SourceProductName=Dare Library
  PaMem_LengthMem2 : DareLib/Dare/getAPI_type  g_funcname=Srvl_GetMemIndexDataU16  g_param=EN_MemIndex_PaMem2_Length  g_type=uint16  g_size=-1
      settings: AttributesFormatString=%<g_funcname>  SourceProductName=Dare Library
  PaMem_LengthMem3 : DareLib/Dare/getAPI_type  g_funcname=Srvl_GetMemIndexDataU16  g_param=EN_MemIndex_PaMem3_Length  g_type=uint16  g_size=-1
      settings: AttributesFormatString=%<g_funcname>  SourceProductName=Dare Library
  PaMem_NapMode : DareLib/Dare/getAPI_type  g_funcname=Rte_GetVfb_NapMode  g_param=""  g_type=uint8  g_enum=enNapMode  g_size=-1
      settings: AttributesFormatString=%<g_funcname>  SourceProductName=Dare Library
  PaMem_PABackSwitch : DareLib/Dare/getAPI_type  g_funcname=Rte_GetVfb_PaBackSwitchCmd  g_param=""  g_type=uint8  g_size=-1
      settings: AttributesFormatString=%<g_funcname>  SourceProductName=Dare Library
  PaMem_PAFrontSwitch : DareLib/Dare/getAPI_type  g_funcname=Rte_GetVfb_PaFrontSwitchCmd  g_param=""  g_type=uint8  g_size=-1
      settings: AttributesFormatString=%<g_funcname>  SourceProductName=Dare Library
  PaMem_PAHeightSwitch : DareLib/Dare/getAPI_type  g_funcname=Rte_GetVfb_PaHeightSwitchCmd  g_param=""  g_type=uint8  g_size=-1
      settings: AttributesFormatString=%<g_funcname>  SourceProductName=Dare Library
  PaMem_PALengthSwitch : DareLib/Dare/getAPI_type  g_funcname=Rte_GetVfb_PaLengthSwitchCmd  g_param=""  g_type=uint8  g_size=-1
      settings: AttributesFormatString=%<g_funcname>  SourceProductName=Dare Library
  PaMem_PaAnyoneLockFaultSts : DareLib/Dare/getAPI_type  g_funcname=Rte_GetVfb_PaAnyoneStallErr  g_param=""  g_type=uint8  g_size=-1
      settings: AttributesFormatString=%<g_funcname>  SourceProductName=Dare Library
  PaMem_PaMemoryConfig : DareLib/Dare/getAPI_type  g_funcname=Srvl_GetMemIndexDataU8  g_param=EN_MemIndex_PaMemoryConfig  g_type=uint8  g_size=-1
      settings: AttributesFormatString=%<g_funcname>  SourceProductName=Dare Library
  PaMem_PowerMode : DareLib/Dare/getAPI_type  g_funcname=Rte_GetVfb_PowerMode  g_param=""  g_type=uint8  g_enum=enPowerModeSts  g_size=-1
      settings: AttributesFormatString=%<g_funcname>  SourceProductName=Dare Library
  PaMem_SeatLearnResult : DareLib/Dare/getAPI_type  g_funcname=Rte_GetVfb_PaLearnResult  g_param=""  g_type=uint8  g_size=-1
      settings: AttributesFormatString=%<g_funcname>  SourceProductName=Dare Library
  PaMem_SeatMemory1Valid : DareLib/Dare/getAPI_type  g_funcname=Srvl_GetMemIndexDataU8  g_param=EN_MemIndex_PaMem1_ValidFlag  g_type=uint8  g_size=-1
      settings: AttributesFormatString=%<g_funcname>  SourceProductName=Dare Library
  PaMem_SeatMemory2Valid : DareLib/Dare/getAPI_type  g_funcname=Srvl_GetMemIndexDataU8  g_param=EN_MemIndex_PaMem2_ValidFlag  g_type=uint8  g_size=-1
      settings: AttributesFormatString=%<g_funcname>  SourceProductName=Dare Library
  PaMem_SeatMemory3Valid : DareLib/Dare/getAPI_type  g_funcname=Srvl_GetMemIndexDataU8  g_param=EN_MemIndex_PaMem3_ValidFlag  g_type=uint8  g_size=-1
      settings: AttributesFormatString=%<g_funcname>  SourceProductName=Dare Library
  PaMem_SpeedLessThan5_Flag : DareLib/Dare/getAPI_type  g_funcname=Rte_GetVfb_SpeedLessThan5_Flag  g_param=""  g_type=uint8  g_size=-1
      settings: AttributesFormatString=%<g_funcname>  SourceProductName=Dare Library
  PaMem_VoltMode : DareLib/Dare/getAPI_type  g_funcname=Rte_GetVfb_VoltMode  g_param=""  g_type=uint8  g_enum=enFinalPowerMode  g_size=-1
      settings: AttributesFormatString=%<g_funcname>  SourceProductName=Dare Library
  PaMem_VoltSatisfy : DareLib/Dare/getAPI_type  g_funcname=Rte_GetVfb_VoltSatisfy  g_param=""  g_type=uint8  g_size=-1
      settings: AttributesFormatString=%<g_funcname>  SourceProductName=Dare Library
  RTE_Signal : Outport
  wires:
  Bus Creator/1 -> RTE_Signal/1  "RTE_Signal"
  PaMem_PAHeightSwitch/1 -> Bus Creator/1  "PaMem_PAHeightSwitch"
  PaMem_PALengthSwitch/1 -> Bus Creator/2  "PaMem_PALengthSwitch"
  PaMem_PABackSwitch/1 -> Bus Creator/3  "PaMem_PABackSwitch"
  PaMem_PAFrontSwitch/1 -> Bus Creator/4  "PaMem_PAFrontSwitch"
  PaMem_HeightAutoRunFlag/1 -> Bus Creator/5  "PaMem_HeightAutoRunFlag"
  PaMem_LengthAutoRunFlag/1 -> Bus Creator/6  "PaMem_LengthAutoRunFlag"
  PaMem_BackAutoRunFlag/1 -> Bus Creator/7  "PaMem_BackAutoRunFlag"
  PaMem_FrontAutoRunFlag/1 -> Bus Creator/8  "PaMem_FrontAutoRunFlag"
  PaMem_HeightLockFault/1 -> Bus Creator/9  "PaMem_HeightLockFault"
  PaMem_LengthLockFault/1 -> Bus Creator/10  "PaMem_LengthLockFault"
  PaMem_BackLockFault/1 -> Bus Creator/11  "PaMem_BackLockFault"
  PaMem_FrontLockFault/1 -> Bus Creator/12  "PaMem_FrontLockFault"
  PaMem_PaAnyoneLockFaultSts/1 -> Bus Creator/13  "PaMem_PaAnyoneLockFaultSts"
  PaMem_DtcAnyoneHallFaultSts/1 -> Bus Creator/14  "PaMem_DtcAnyoneHallFaultSts"
  PaMem_AnyoneRelayFaultSts/1 -> Bus Creator/15  "PaMem_AnyoneRelayFaultSts"
  PaMem_Gear_PN_FlagOut/1 -> Bus Creator/16  "PaMem_Gear_PN_FlagOut"
  PaMem_HeightHallPosi/1 -> Bus Creator/17  "PaMem_HeightHallPosi"
  PaMem_LengthHallPosi/1 -> Bus Creator/18  "PaMem_LengthHallPosi"
  PaMem_BackHallPosi/1 -> Bus Creator/19  "PaMem_BackHallPosi"
  PaMem_FrontHallPosi/1 -> Bus Creator/20  "PaMem_FrontHallPosi"
  PaMem_HeightMem1/1 -> Bus Creator/21  "PaMem_HeightMem1"
  PaMem_LengthMem1/1 -> Bus Creator/22  "PaMem_LengthMem1"
  PaMem_BackMem1/1 -> Bus Creator/23  "PaMem_BackMem1"
  PaMem_FrontMem1/1 -> Bus Creator/24  "PaMem_FrontMem1"
  PaMem_HeightMem2/1 -> Bus Creator/25  "PaMem_HeightMem2"
  PaMem_LengthMem2/1 -> Bus Creator/26  "PaMem_LengthMem2"
  PaMem_BackMem2/1 -> Bus Creator/27  "PaMem_BackMem2"
  PaMem_FrontMem2/1 -> Bus Creator/28  "PaMem_FrontMem2"
  PaMem_HeightMem3/1 -> Bus Creator/29  "PaMem_HeightMem3"
  PaMem_LengthMem3/1 -> Bus Creator/30  "PaMem_LengthMem3"
  PaMem_BackMem3/1 -> Bus Creator/31  "PaMem_BackMem3"
  PaMem_FrontMem3/1 -> Bus Creator/32  "PaMem_FrontMem3"
  PaMem_FRSeatPosMsg/1 -> Bus Creator/33  "PaMem_FRSeatPosMsg"
  PaMem_SeatMemory1Valid/1 -> Bus Creator/34  "PaMem_SeatMemory1Valid"
  PaMem_SeatMemory2Valid/1 -> Bus Creator/35  "PaMem_SeatMemory2Valid"
  PaMem_SeatMemory3Valid/1 -> Bus Creator/36  "PaMem_SeatMemory3Valid"
  PaMem_PaMemoryConfig/1 -> Bus Creator/37  "PaMem_PaMemoryConfig"
  PaMem_AdjustEnable/1 -> Bus Creator/38  "PaMem_AdjustEnable"
  PaMem_IVI_FRSeatMemSet1/1 -> Bus Creator/39  "PaMem_IVI_FRSeatMemSet1"
  PaMem_IVI_FRSeatMemSet2/1 -> Bus Creator/40  "PaMem_IVI_FRSeatMemSet2"
  PaMem_IVI_FRSeatMemSet3/1 -> Bus Creator/41  "PaMem_IVI_FRSeatMemSet3"
  PaMem_SpeedLessThan5_Flag/1 -> Bus Creator/42  "PaMem_SpeedLessThan5_Flag"
  PaMem_CurrentMoveType/1 -> Bus Creator/43  "PaMem_CurrentMoveType"
  PaMem_SeatLearnResult/1 -> Bus Creator/44  "PaMem_SeatLearnResult"
  PaMem_NapMode/1 -> Bus Creator/45  "PaMem_NapMode"
  PaMem_GetRecoverDefaultFlag/1 -> Bus Creator/46  "PaMem_GetRecoverDefaultFlag"
  PaMem_VoltMode/1 -> Bus Creator/47  "PaMem_VoltMode"
  PaMem_PowerMode/1 -> Bus Creator/48  "PaMem_PowerMode"
  PaMem_VoltSatisfy/1 -> Bus Creator/49  "PaMem_VoltSatisfy"

== system Appl_PaMemory_CtrlModel/LogicCtrl/LocalAdjustCtrl/MemoryCall/GetCanSendEvent ==
  f : TriggerPort  TriggerType=function-call  VariantControl=(inherit)
      settings: CopyFcn=Stateflow.SLINSF.SimulinkMan.removeBlockPreDeleteFcn  PreDeleteFcn=Stateflow.SLINSF.SimulinkMan.unsafePredeleteFcn
  DrMem_FrontHallPosi : DareLib/Dare/getAPI_type  g_funcname=Rte_GetCanEventSendTimes_0x3B2  g_param=""  g_type=uint16  g_size=-1
      settings: AttributesFormatString=%<g_funcname>  SourceProductName=Dare Library
  Out1 : Outport
  wires:
  DrMem_FrontHallPosi/1 -> Out1/1

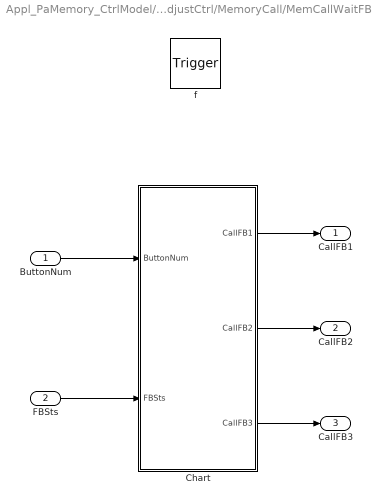
== system Appl_PaMemory_CtrlModel/LogicCtrl/LocalAdjustCtrl/MemoryCall/MemCallWaitFBFunc ==
  ButtonNum : Inport
  FBSts : Inport  Port=2
  f : TriggerPort  TriggerType=function-call  VariantControl=(inherit)
      settings: CopyFcn=Stateflow.SLINSF.SimulinkMan.removeBlockPreDeleteFcn  PreDeleteFcn=Stateflow.SLINSF.SimulinkMan.unsafePredeleteFcn
  Chart : Stateflow chart  TreatAsAtomicUnit=on
  CallFB1 : Outport
  CallFB2 : Outport  Port=2
  CallFB3 : Outport  Port=3
  wires:
  ButtonNum/1 -> Chart/1(ButtonNum)
  FBSts/1 -> Chart/2(FBSts)
  Chart/1(CallFB1) -> CallFB1/1
  Chart/2(CallFB2) -> CallFB2/1
  Chart/3(CallFB3) -> CallFB3/1

== system Appl_PaMemory_CtrlModel/LogicCtrl/LocalAdjustCtrl/MemoryCall/SetCanSendEvent ==
  In1 : Inport
  f : TriggerPort  TriggerType=function-call  VariantControl=(inherit)
      settings: CopyFcn=Stateflow.SLINSF.SimulinkMan.removeBlockPreDeleteFcn  PreDeleteFcn=Stateflow.SLINSF.SimulinkMan.unsafePredeleteFcn
  DrMemO_SeatMem1StsFb : DareLib/Dare/setAPI_type  g_funcname=Rte_SetCanEvent_0x3B2  g_param=""  g_type=uint16  g_size=-1
      settings: AttributesFormatString=%<g_funcname>  SourceProductName=Dare Library
  wires:
  In1/1 -> DrMemO_SeatMem1StsFb/1

== system Appl_PaMemory_CtrlModel/LogicCtrl/LocalAdjustCtrl/MemoryCall/SetCanSendFRSeatMem1Sts ==
  In1 : Inport
  f : TriggerPort  TriggerType=function-call  VariantControl=(inherit)
      settings: CopyFcn=Stateflow.SLINSF.SimulinkMan.removeBlockPreDeleteFcn  PreDeleteFcn=Stateflow.SLINSF.SimulinkMan.unsafePredeleteFcn
  DrMemO_SeatMem1StsFb : DareLib/Dare/setAPI_type  g_funcname=CanTx_0x3B2_DSM1_FRSeatMem1Sts  g_param=""  g_type=uint16  g_size=-1
      settings: AttributesFormatString=%<g_funcname>  SourceProductName=Dare Library
  wires:
  In1/1 -> DrMemO_SeatMem1StsFb/1

== system Appl_PaMemory_CtrlModel/LogicCtrl/LocalAdjustCtrl/MemoryCall/SetCanSendFRSeatMem2Sts ==
  In1 : Inport
  f : TriggerPort  TriggerType=function-call  VariantControl=(inherit)
      settings: CopyFcn=Stateflow.SLINSF.SimulinkMan.removeBlockPreDeleteFcn  PreDeleteFcn=Stateflow.SLINSF.SimulinkMan.unsafePredeleteFcn
  DrMemO_SeatMem1StsFb : DareLib/Dare/setAPI_type  g_funcname=CanTx_0x3B2_DSM2_FRSeatMem2Sts  g_param=""  g_type=uint16  g_size=-1
      settings: AttributesFormatString=%<g_funcname>  SourceProductName=Dare Library
  wires:
  In1/1 -> DrMemO_SeatMem1StsFb/1

== system Appl_PaMemory_CtrlModel/LogicCtrl/LocalAdjustCtrl/MemoryCall/SetCanSendFRSeatMem3Sts ==
  In1 : Inport
  f : TriggerPort  TriggerType=function-call  VariantControl=(inherit)
      settings: CopyFcn=Stateflow.SLINSF.SimulinkMan.removeBlockPreDeleteFcn  PreDeleteFcn=Stateflow.SLINSF.SimulinkMan.unsafePredeleteFcn
  DrMemO_SeatMem1StsFb : DareLib/Dare/setAPI_type  g_funcname=CanTx_0x3B2_DSM2_FRSeatMem3Sts  g_param=""  g_type=uint16  g_size=-1
      settings: AttributesFormatString=%<g_funcname>  SourceProductName=Dare Library
  wires:
  In1/1 -> DrMemO_SeatMem1StsFb/1

== system Appl_PaMemory_CtrlModel/LogicCtrl/LocalAdjustCtrl/MemoryRemindLogic/GetCanSendEvent ==
  f : TriggerPort  TriggerType=function-call  VariantControl=(inherit)
      settings: CopyFcn=Stateflow.SLINSF.SimulinkMan.removeBlockPreDeleteFcn  PreDeleteFcn=Stateflow.SLINSF.SimulinkMan.unsafePredeleteFcn
  DrMem_FrontHallPosi : DareLib/Dare/getAPI_type  g_funcname=Rte_GetCanEventSendTimes_0x3B2  g_param=""  g_type=uint16  g_size=-1
      settings: AttributesFormatString=%<g_funcname>  SourceProductName=Dare Library
  Out1 : Outport
  wires:
  DrMem_FrontHallPosi/1 -> Out1/1

== system Appl_PaMemory_CtrlModel/LogicCtrl/LocalAdjustCtrl/MemoryRemindLogic/SetCanSendEvent ==
  In1 : Inport
  f : TriggerPort  TriggerType=function-call  VariantControl=(inherit)
      settings: CopyFcn=Stateflow.SLINSF.SimulinkMan.removeBlockPreDeleteFcn  PreDeleteFcn=Stateflow.SLINSF.SimulinkMan.unsafePredeleteFcn
  DrMemO_SeatMem1StsFb : DareLib/Dare/setAPI_type  g_funcname=Rte_SetCanEvent_0x3B2  g_param=""  g_type=uint16  g_size=-1
      settings: AttributesFormatString=%<g_funcname>  SourceProductName=Dare Library
  wires:
  In1/1 -> DrMemO_SeatMem1StsFb/1

== system Appl_PaMemory_CtrlModel/LogicCtrl/LocalAdjustCtrl/MemoryRemindLogic/SetCanSendFRSeatPosMsg ==
  In1 : Inport
  f : TriggerPort  TriggerType=function-call  VariantControl=(inherit)
      settings: CopyFcn=Stateflow.SLINSF.SimulinkMan.removeBlockPreDeleteFcn  PreDeleteFcn=Stateflow.SLINSF.SimulinkMan.unsafePredeleteFcn
  DrMemO_SeatMem1StsFb : DareLib/Dare/setAPI_type  g_funcname=CanTx_0x3B2_DSM_FRSeatPosMsg  g_param=""  g_type=uint16  g_size=-1
      settings: AttributesFormatString=%<g_funcname>  SourceProductName=Dare Library
  wires:
  In1/1 -> DrMemO_SeatMem1StsFb/1

== system Appl_PaMemory_CtrlModel/LogicCtrl/LocalAdjustCtrl/MemoryRemindLogic/WriteFLSeatPosMsg ==
  Sts : Inport
  f : TriggerPort  TriggerType=function-call  VariantControl=(inherit)
      settings: CopyFcn=Stateflow.SLINSF.SimulinkMan.removeBlockPreDeleteFcn  PreDeleteFcn=Stateflow.SLINSF.SimulinkMan.unsafePredeleteFcn
  DrMemO_SeatBackPosiReq : DareLib/Dare/setAPI_type  g_funcname=Srvl_SetMemIndexDataU8  g_param=EN_MemIndex_FRSeatPosMsg  g_type=uint16  g_size=-1
      settings: AttributesFormatString=%<g_funcname>  SourceProductName=Dare Library
  wires:
  Sts/1 -> DrMemO_SeatBackPosiReq/1

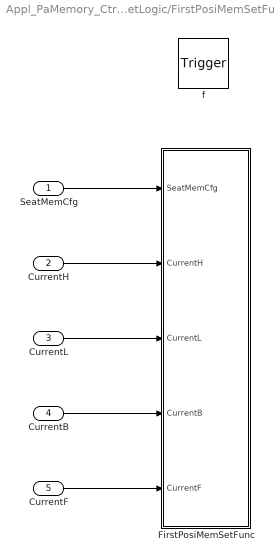
== system Appl_PaMemory_CtrlModel/LogicCtrl/LocalAdjustCtrl/MemorySetLogic/FirstPosiMemSetFunc ==
  SeatMemCfg : Inport
  CurrentH : Inport  Port=2
  CurrentL : Inport  Port=3
  CurrentB : Inport  Port=4
  CurrentF : Inport  Port=5
  f : TriggerPort  TriggerType=function-call  VariantControl=(inherit)
      settings: CopyFcn=Stateflow.SLINSF.SimulinkMan.removeBlockPreDeleteFcn  PreDeleteFcn=Stateflow.SLINSF.SimulinkMan.unsafePredeleteFcn
  FirstPosiMemSetFunc : Stateflow chart  TreatAsAtomicUnit=on
  wires:
  CurrentH/1 -> FirstPosiMemSetFunc/2(CurrentH)
  CurrentL/1 -> FirstPosiMemSetFunc/3(CurrentL)
  SeatMemCfg/1 -> FirstPosiMemSetFunc/1(SeatMemCfg)
  CurrentB/1 -> FirstPosiMemSetFunc/4(CurrentB)
  CurrentF/1 -> FirstPosiMemSetFunc/5(CurrentF)

== system Appl_PaMemory_CtrlModel/LogicCtrl/LocalAdjustCtrl/MemorySetLogic/GetCanSendEvent ==
  f : TriggerPort  TriggerType=function-call  VariantControl=(inherit)
      settings: CopyFcn=Stateflow.SLINSF.SimulinkMan.removeBlockPreDeleteFcn  PreDeleteFcn=Stateflow.SLINSF.SimulinkMan.unsafePredeleteFcn
  DrMem_FrontHallPosi : DareLib/Dare/getAPI_type  g_funcname=Rte_GetCanEventSendTimes_0x3B2  g_param=""  g_type=uint16  g_size=-1
      settings: AttributesFormatString=%<g_funcname>  SourceProductName=Dare Library
  Out1 : Outport
  wires:
  DrMem_FrontHallPosi/1 -> Out1/1

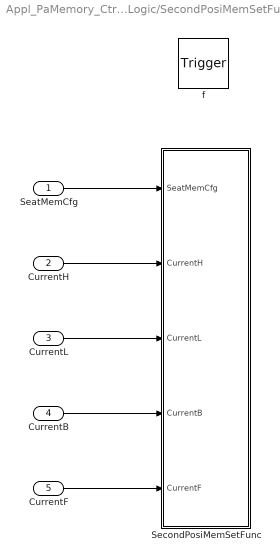
== system Appl_PaMemory_CtrlModel/LogicCtrl/LocalAdjustCtrl/MemorySetLogic/SecondPosiMemSetFunc ==
  SeatMemCfg : Inport
  CurrentH : Inport  Port=2
  CurrentL : Inport  Port=3
  CurrentB : Inport  Port=4
  CurrentF : Inport  Port=5
  f : TriggerPort  TriggerType=function-call  VariantControl=(inherit)
      settings: CopyFcn=Stateflow.SLINSF.SimulinkMan.removeBlockPreDeleteFcn  PreDeleteFcn=Stateflow.SLINSF.SimulinkMan.unsafePredeleteFcn
  SecondPosiMemSetFunc : Stateflow chart  TreatAsAtomicUnit=on
  wires:
  CurrentH/1 -> SecondPosiMemSetFunc/2(CurrentH)
  CurrentL/1 -> SecondPosiMemSetFunc/3(CurrentL)
  SeatMemCfg/1 -> SecondPosiMemSetFunc/1(SeatMemCfg)
  CurrentB/1 -> SecondPosiMemSetFunc/4(CurrentB)
  CurrentF/1 -> SecondPosiMemSetFunc/5(CurrentF)

== system Appl_PaMemory_CtrlModel/LogicCtrl/LocalAdjustCtrl/MemorySetLogic/SetCanSendEvent ==
  In1 : Inport
  f : TriggerPort  TriggerType=function-call  VariantControl=(inherit)
      settings: CopyFcn=Stateflow.SLINSF.SimulinkMan.removeBlockPreDeleteFcn  PreDeleteFcn=Stateflow.SLINSF.SimulinkMan.unsafePredeleteFcn
  DrMemO_SeatMem1StsFb : DareLib/Dare/setAPI_type  g_funcname=Rte_SetCanEvent_0x3B2  g_param=""  g_type=uint16  g_size=-1
      settings: AttributesFormatString=%<g_funcname>  SourceProductName=Dare Library
  wires:
  In1/1 -> DrMemO_SeatMem1StsFb/1

== system Appl_PaMemory_CtrlModel/LogicCtrl/LocalAdjustCtrl/MemorySetLogic/SetCanSendMemStsAndMsg ==
  In1 : Inport
  f : TriggerPort  TriggerType=function-call  VariantControl=(inherit)
      settings: CopyFcn=Stateflow.SLINSF.SimulinkMan.removeBlockPreDeleteFcn  PreDeleteFcn=Stateflow.SLINSF.SimulinkMan.unsafePredeleteFcn
  DrMemO_SeatMem1StsFb : DareLib/Dare/setAPI_type  g_funcname=CanTx_0x3B2_DSM_FRSeatMemStsAndMsg  g_param=""  g_type=uint16  g_size=-1
      settings: AttributesFormatString=%<g_funcname>  SourceProductName=Dare Library
  wires:
  In1/1 -> DrMemO_SeatMem1StsFb/1

== system Appl_PaMemory_CtrlModel/LogicCtrl/LocalAdjustCtrl/MemorySetLogic/ThirdPosiMemSetFunc ==
  SeatMemCfg : Inport
  CurrentH : Inport  Port=2
  CurrentL : Inport  Port=3
  CurrentB : Inport  Port=4
  CurrentF : Inport  Port=5
  f : TriggerPort  TriggerType=function-call  VariantControl=(inherit)
      settings: CopyFcn=Stateflow.SLINSF.SimulinkMan.removeBlockPreDeleteFcn  PreDeleteFcn=Stateflow.SLINSF.SimulinkMan.unsafePredeleteFcn
  ThirdPosiMemSetFunc : Stateflow chart  TreatAsAtomicUnit=on
  wires:
  CurrentH/1 -> ThirdPosiMemSetFunc/2(CurrentH)
  CurrentL/1 -> ThirdPosiMemSetFunc/3(CurrentL)
  SeatMemCfg/1 -> ThirdPosiMemSetFunc/1(SeatMemCfg)
  CurrentB/1 -> ThirdPosiMemSetFunc/4(CurrentB)
  CurrentF/1 -> ThirdPosiMemSetFunc/5(CurrentF)

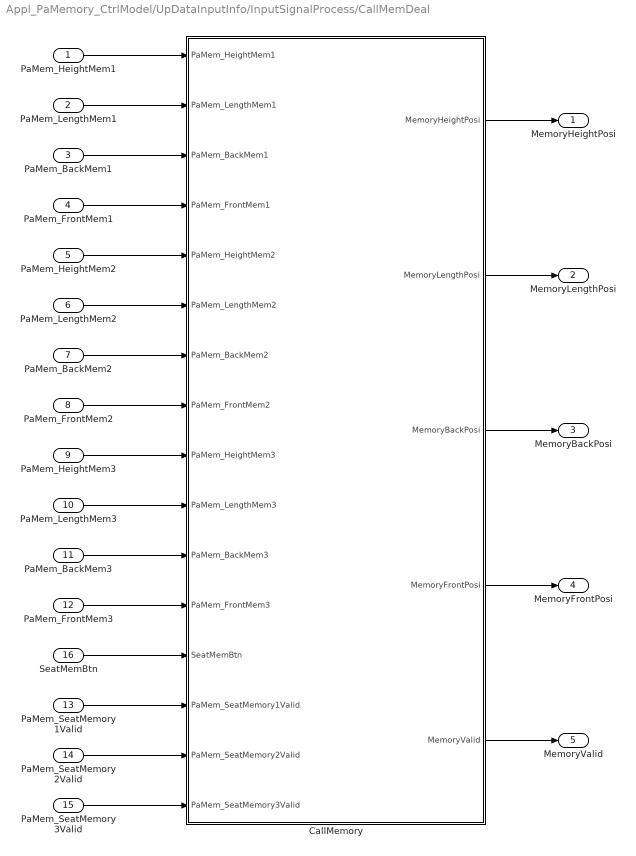
== system Appl_PaMemory_CtrlModel/UpDataInputInfo/InputSignalProcess/CallMemDeal ==
  PaMem_HeightMem1 : Inport
  PaMem_LengthMem1 : Inport  Port=2
  PaMem_BackMem1 : Inport  Port=3
  PaMem_FrontMem1 : Inport  Port=4
  PaMem_HeightMem2 : Inport  Port=5
  PaMem_LengthMem2 : Inport  Port=6
  PaMem_BackMem2 : Inport  Port=7
  PaMem_FrontMem2 : Inport  Port=8
  PaMem_HeightMem3 : Inport  Port=9
  PaMem_LengthMem3 : Inport  Port=10
  PaMem_BackMem3 : Inport  Port=11
  PaMem_FrontMem3 : Inport  Port=12
  PaMem_SeatMemory1Valid : Inport  Port=13
  PaMem_SeatMemory2Valid : Inport  Port=14
  PaMem_SeatMemory3Valid : Inport  Port=15
  SeatMemBtn : Inport  Port=16
  CallMemory : Stateflow chart  TreatAsAtomicUnit=on
  MemoryHeightPosi : Outport
  MemoryLengthPosi : Outport  Port=2
  MemoryBackPosi : Outport  Port=3
  MemoryFrontPosi : Outport  Port=4
  MemoryValid : Outport  Port=5
  wires:
  PaMem_LengthMem1/1 -> CallMemory/2(PaMem_LengthMem1)
  PaMem_BackMem1/1 -> CallMemory/3(PaMem_BackMem1)
  PaMem_HeightMem1/1 -> CallMemory/1(PaMem_HeightMem1)
  PaMem_FrontMem1/1 -> CallMemory/4(PaMem_FrontMem1)
  PaMem_HeightMem2/1 -> CallMemory/5(PaMem_HeightMem2)
  PaMem_LengthMem2/1 -> CallMemory/6(PaMem_LengthMem2)
  PaMem_BackMem2/1 -> CallMemory/7(PaMem_BackMem2)
  PaMem_FrontMem2/1 -> CallMemory/8(PaMem_FrontMem2)
  PaMem_HeightMem3/1 -> CallMemory/9(PaMem_HeightMem3)
  PaMem_LengthMem3/1 -> CallMemory/10(PaMem_LengthMem3)
  PaMem_BackMem3/1 -> CallMemory/11(PaMem_BackMem3)
  SeatMemBtn/1 -> CallMemory/13(SeatMemBtn)
  PaMem_FrontMem3/1 -> CallMemory/12(PaMem_FrontMem3)
  CallMemory/1(MemoryHeightPosi) -> MemoryHeightPosi/1
  CallMemory/3(MemoryBackPosi) -> MemoryBackPosi/1
  CallMemory/4(MemoryFrontPosi) -> MemoryFrontPosi/1
  CallMemory/2(MemoryLengthPosi) -> MemoryLengthPosi/1
  CallMemory/5(MemoryValid) -> MemoryValid/1
  PaMem_SeatMemory3Valid/1 -> CallMemory/16(PaMem_SeatMemory3Valid)
  PaMem_SeatMemory2Valid/1 -> CallMemory/15(PaMem_SeatMemory2Valid)
  PaMem_SeatMemory1Valid/1 -> CallMemory/14(PaMem_SeatMemory1Valid)
